simulink model "NodoseNeuron"  (Simulink 7.0)
settings: Solver=ode45  StartTime=0.0  StopTime=1000  MaxStep=20  RelTol=1e-3
InitFcn:
  | T=310.0;       % K
  | R=8.3145;     % J/mole/K or V*C/mol/K
  | F=96485.0;    % C/mole
  | Nai=8.9;         % mM
  | Nao=154;       % mM
  | Ki=145;           % mM
  | Ko=5.4;           % mM
  | Cai=0.0001;    %mM
  | Cao=2.0;         %mM
  | %Cli Clo
  | %Hi Ho
  | %Cli Clo
  | 
  | ENa=R*T/F*log(Nao/Nai)*1000;    % mV
  | EK=R*T/F*log(Ko/Ki)*1000;           % mM
  | ECa=R*T/2/F*log(Cao/Cai)*1000; % mV
  | %EH=R*T/F*log(Ho/Hi)*1000;
  | %ECl=R*T//F*log(Clo/Cli)*1000;
  | 
  | tauCa=4511.0;   % ms
  | nBi=0.004;         % mM (concentration of Ca2+ buffer) * (number of Ca2+ binding sights)
  | Voli=0.0127;      % nl
  | Vols=0.00146;   % nl
  | 
  | ICaP=0.0243;          % nA
  | INaK=0.275;            % nA
  | DNaCa=0.0036;      % 1/mM^4
  | KNaCa=0.000036;  % nA/mM^4
  | KMCaP=0.0005;     % mM
  | KMNa=5.46;           % mM
  | KMK=0.621;            % mM
  | kU=100.0;               % 1/mM/ms
  | kR=0.238;               % 1/ms
undefined symbols (not defined in the file): sigbuilder_block
settings Model: Creator=Vlad  LastModifiedBy=snitsarevv  ExtModeAutoUpdateStatusClock=off  TunableVars=gA,gBCa,gBNa,gCan,gCat,gD,gK,gKCa,gNaf,gNas  TunableVarsStorageClass=Auto,Auto,Auto,Auto,Auto,Auto,Auto,Auto,Auto,Auto  TunableVarsTypeQualifier=,,,,,,,,,  BufferReuse=off
settings SolverCC: ZeroCrossControl=DisableAll
settings DataIOCC: ExternalInput=[t u]  LimitDataPoints=off
settings OptimizationCC: InlineParams=on  OptimizeBlockIOStorage=off  BufferReuse=off  ExpressionFolding=off  LocalBlockOutputs=off
settings DebuggingCC: SaveWithParameterizedLinksMsg=none
settings GRTTargetCC: TargetFcnLib=ansi_tfl_tmw.mat

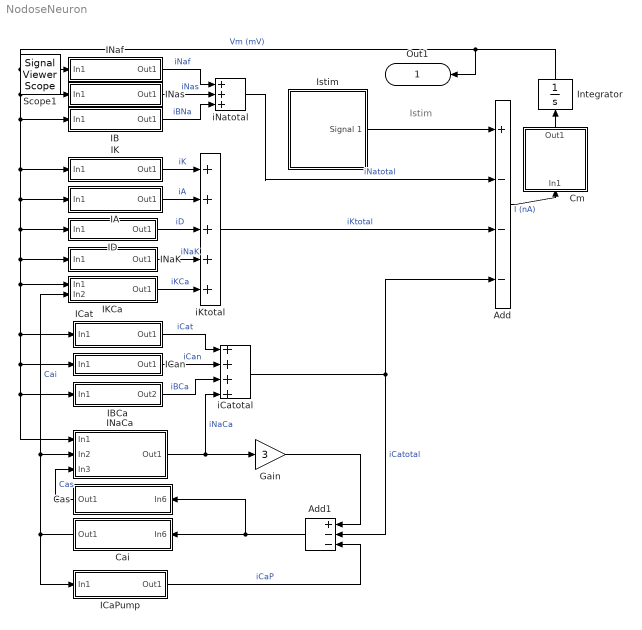
== system NodoseNeuron ==
  note: Istim
  Add : Sum  Inputs=+---  OutDataType=sfix(16)  OutScaling=2^-10
  Add1 : Sum  Orientation=left  Inputs=+--  OutDataType=sfix(16)  OutScaling=2^-10
  Cai : Subsystem  Orientation=left
  Cas : Subsystem  Orientation=left
  Cm : Subsystem  Orientation=up  mask{Cm=32.5}
      mask help: Cm=32.5 pF
  Gain : Gain  Gain=3  ParameterDataType=sfix(16)  ParameterScaling=2^0  OutDataType=sfix(16)  OutScaling=2^0
  IA : Subsystem  mask{gA=0.035}
      mask help: gA=0.035 microS
      mask init:
      | %gA=0.035 in SK model
  IB : Subsystem  mask{gBNa=0.000325}
      mask help: gBNa=0.000325 microS
  IBCa : Subsystem  mask{gBCa=0.000085}
      mask help: gBCa=0.000085 microS
  ICaPump : Subsystem
  ICan : Subsystem  mask{gCan=0.001}
      mask help: gCan=0.001 microS
  ICat : Subsystem  mask{gCat=0.00035}
      mask help: gCat=0.00035 microS
  ID : Subsystem  mask{gD=0.01}
      mask help: gD=0.01 microS
  IK : Subsystem  mask{gK=0.0055}
      mask help: gK=0.0055 microS
  IKCa : Subsystem  mask{gKCa=0.0065}
      mask help: gKCa=0.0065 microS
  INaCa : Subsystem
  INaK : Subsystem
  INaf : Subsystem  mask{gNaf=2.05}
      mask help: gNaf=2.05 microS
  INas : Subsystem  mask{gNas=0.00001}
      mask help: gNas=0.00001 microS
  Integrator : Integrator  Orientation=up  InitialCondition=-56.34  UpperSaturationLimit=100  LowerSaturationLimit=-100
  Istim : Subsystem  Tag=STV Subsys  LoadFcn=sigbuilder_block('load');  StartFcn=sigbuilder_block('start');  StopFcn=sigbuilder_block('stop');  ClipboardFcn=sigbuilder_block('clipboard');  mask(Sigbuilder block){}
      mask help: Sigbuilder GUI
      mask init:
      | if ~strcmp(get_param(bdroot(gcbh),'SimulationStatus'),'stopped') tuvar = sigbuilder_block('maskInit'); end
      settings: CopyFcn=sigbuilder_block('copy');  DeleteFcn=sigbuilder_block('delete');  ModelCloseFcn=sigbuilder_block('modelClose');  PreSaveFcn=sigbuilder_block('preSave');  NameChangeFcn=sigbuilder_block('namechange');  OpenFcn=sigbuilder_block('open',[293.25 508.5 663.75 206.25 ]);  CloseFcn=sigbuilder_block('close');
      mask Display: plot(0,0,100,100,[10,10,40,40,10],[80,20,20,80,80],[40,10],[50,50], [40,27,10],[65,72,56],[40,25,25,10],[28,28,43,43]);
  iCatotal : Sum  Inputs=++++  OutDataType=sfix(16)  OutScaling=2^-10
  iKtotal : Sum  Inputs=+++++  OutDataType=sfix(16)  OutScaling=2^-10
  iNatotal : Sum  Inputs=+++  OutDataType=sfix(16)  OutScaling=2^-10
  Out1 : Outport  Orientation=left  OutDataType=sfix(16)  OutScaling=2^0
  Scope1 : SignalViewerScope  IOType=viewer  LegendLocations="567.3333           436            97      20.33333"  RefreshTime=0.035000
      settings: ShowLegends=on  TimeRange=1000  YMin=-80  YMax=80
  wires:
  Cm/1(Out1) -> Integrator/1
  Add/1 -> Cm/1(In1)  "I (nA)"
  INaf/1(Out1) -> iNatotal/1  "iNaf"
  INas/1(Out1) -> iNatotal/2  "iNas"
  IK/1(Out1) -> iKtotal/1  "iK"
  IA/1(Out1) -> iKtotal/2  "iA"
  ID/1(Out1) -> iKtotal/3  "iD"
  INaK/1(Out1) -> iKtotal/4  "iNaK"
  Cas/1(Out1) -> INaCa/3(In3)  "Cas"
  Cai/1(Out1) -> INaCa/2(In2), IKCa/2(In2), ICaPump/1(In1)  "Cai"
  IKCa/1(Out1) -> iKtotal/5  "iKCa"
  IB/1(Out1) -> iNatotal/3  "iBNa"
  ICat/1(Out1) -> iCatotal/1  "iCat"
  ICan/1(Out1) -> iCatotal/2  "iCan"
  iCatotal/1 -> Add1/2, Add/4  "iCatotal"
  ICaPump/1(Out1) -> Add1/3  "iCaP"
  INaCa/1(Out1) -> iCatotal/4, Gain/1  "iNaCa"
  Add1/1 -> Cas/1(In6), Cai/1(In6)
  Gain/1 -> Add1/1
  iKtotal/1 -> Add/3  "iKtotal"
  iNatotal/1 -> Add/2  "iNatotal"
  Integrator/1 -> Out1/1, INaf/1(In1), INas/1(In1), IB/1(In1), IA/1(In1), ID/1(In1), INaK/1(In1), IBCa/1(In1), INaCa/1(In1), ICan/1(In1), ICat/1(In1), IKCa/1(In1), IK/1(In1)  "Vm (mV)"
  Istim/1(Signal 1) -> Add/1
  IBCa/1(Out2) -> iCatotal/3  "iBCa"

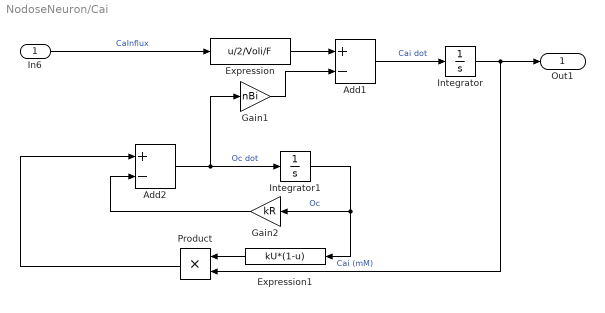
== system NodoseNeuron/Cai ==
  In6 : Inport  OutDataType=sfix(16)  OutScaling=2^0
  Add1 : Sum  Inputs=+-  OutDataType=sfix(16)  OutScaling=2^-10
  Add2 : Sum  Inputs=+-  OutDataType=sfix(16)  OutScaling=2^-10
  Expression : Fcn  Expr=u/2/Voli/F
  Expression1 : Fcn  Orientation=left  Expr=kU*(1-u)
  Gain1 : Gain  Gain=nBi  ParameterDataType=sfix(16)  ParameterScaling=2^0  OutDataType=sfix(16)  OutScaling=2^0
  Gain2 : Gain  Orientation=left  Gain=kR  ParameterDataType=sfix(16)  ParameterScaling=2^0  OutDataType=sfix(16)  OutScaling=2^0
  Integrator : Integrator  InitialCondition=0.00008424  LimitOutput=on  UpperSaturationLimit=0.001  LowerSaturationLimit=0
  Integrator1 : Integrator  InitialCondition=0.03418  LimitOutput=on  UpperSaturationLimit=1  LowerSaturationLimit=0
  Product : Product  Orientation=left  OutDataType=sfix(16)  OutScaling=2^0  RndMeth=Zero
  Out1 : Outport  OutDataType=sfix(16)  OutScaling=2^0
  wires:
  Add1/1 -> Integrator/1  "Cai dot"
  Integrator/1 -> Out1/1, Product/2  "Cai (mM)"
  In6/1 -> Expression/1  "CaInflux"
  Expression/1 -> Add1/1
  Add2/1 -> Integrator1/1, Gain1/1  "Oc dot"
  Gain1/1 -> Add1/2
  Integrator1/1 -> Expression1/1, Gain2/1  "Oc"
  Expression1/1 -> Product/1
  Product/1 -> Add2/1
  Gain2/1 -> Add2/2

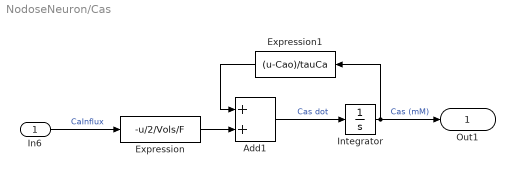
== system NodoseNeuron/Cas ==
  In6 : Inport  OutDataType=sfix(16)  OutScaling=2^0
  Add1 : Sum  OutDataType=sfix(16)  OutScaling=2^-10
  Expression : Fcn  Expr=-u/2/Vols/F
  Expression1 : Fcn  Orientation=left  Expr=(u-Cao)/tauCa
  Integrator : Integrator  InitialCondition=1.7131  LimitOutput=on  UpperSaturationLimit=2  LowerSaturationLimit=0
  Out1 : Outport  OutDataType=sfix(16)  OutScaling=2^0
  wires:
  In6/1 -> Expression/1  "CaInflux"
  Integrator/1 -> Expression1/1, Out1/1  "Cas (mM)"
  Expression1/1 -> Add1/1
  Add1/1 -> Integrator/1  "Cas dot"
  Expression/1 -> Add1/2

== system NodoseNeuron/Cm ==
  In1 : Inport  Orientation=up  OutDataType=sfix(16)  OutScaling=2^0
  Cm : Fcn  Orientation=up  Expr=u/Cm*1000.0
  Out1 : Outport  Orientation=up  OutDataType=sfix(16)  OutScaling=2^0
  wires:
  Cm/1 -> Out1/1  "Vm dot"
  In1/1 -> Cm/1

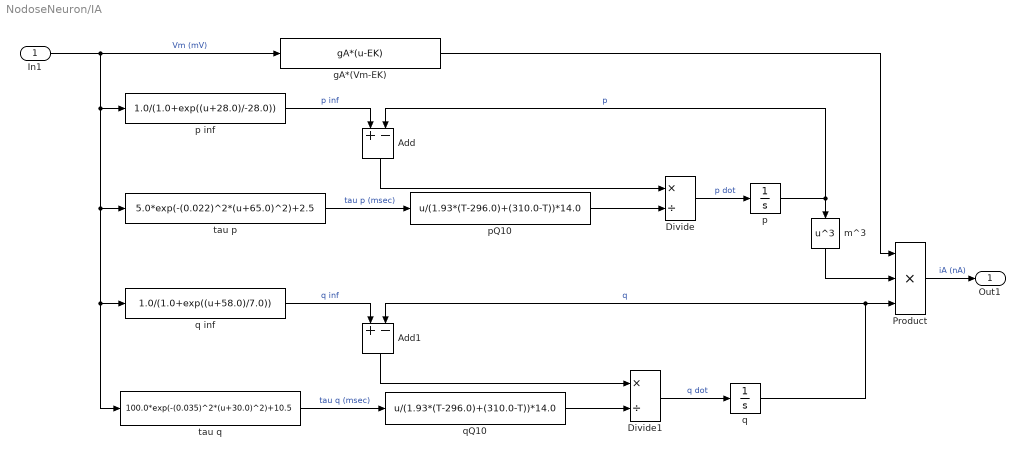
== system NodoseNeuron/IA ==
  In1 : Inport  OutDataType=sfix(16)  OutScaling=2^0
  Add : Sum  Orientation=down  Inputs=+-  OutDataType=sfix(16)  OutScaling=2^-10
  Add1 : Sum  Orientation=down  Inputs=+-  OutDataType=sfix(16)  OutScaling=2^-10
  Divide : Product  Inputs=*/  OutDataType=sfix(16)  OutScaling=2^-10
  Divide1 : Product  Inputs=*/  OutDataType=sfix(16)  OutScaling=2^-10
  Product : Product  Inputs=3  OutDataType=sfix(16)  OutScaling=2^0  RndMeth=Zero
  gA*(Vm-EK) : Fcn  Expr=gA*(u-EK)
  m^3 : Fcn  Orientation=down  Expr=u^3
  p : Integrator  InitialCondition=0.2866  LimitOutput=on  UpperSaturationLimit=1  LowerSaturationLimit=0
  p inf : Fcn  Expr=1.0/(1.0+exp((u+28.0)/-28.0))
  pQ10 : Fcn  Expr=u/(1.93*(T-296.0)+(310.0-T))*14.0
  q : Integrator  InitialCondition=0.3455  LimitOutput=on  UpperSaturationLimit=1  LowerSaturationLimit=0
  q inf : Fcn  Expr=1.0/(1.0+exp((u+58.0)/7.0))
  qQ10 : Fcn  Expr=u/(1.93*(T-296.0)+(310.0-T))*14.0
  tau p : Fcn  Expr=5.0*exp(-(0.022)^2*(u+65.0)^2)+2.5
  tau q : Fcn  Expr=100.0*exp(-(0.035)^2*(u+30.0)^2)+10.5
  Out1 : Outport  OutDataType=sfix(16)  OutScaling=2^0  InitialOutput=0
  wires:
  In1/1 -> q inf/1, tau q/1, tau p/1, p inf/1, gA*(Vm-EK)/1  "Vm (mV)"
  p inf/1 -> Add/1  "p inf"
  p/1 -> m^3/1, Add/2  "p"
  tau p/1 -> pQ10/1  "tau p (msec)"
  Add/1 -> Divide/1
  Divide/1 -> p/1  "p dot"
  q inf/1 -> Add1/1  "q inf"
  Divide1/1 -> q/1  "q dot"
  Add1/1 -> Divide1/1
  tau q/1 -> qQ10/1  "tau q (msec)"
  q/1 -> Add1/2, Product/3  "q"
  Product/1 -> Out1/1  "iA (nA)"
  pQ10/1 -> Divide/2
  qQ10/1 -> Divide1/2
  gA*(Vm-EK)/1 -> Product/1
  m^3/1 -> Product/2

== system NodoseNeuron/IB ==
  In1 : Inport  OutDataType=sfix(16)  OutScaling=2^0
  IBNa : Fcn  Expr=gBNa*(u-ENa)
  Out1 : Outport  OutDataType=sfix(16)  OutScaling=2^0  InitialOutput=0
  wires:
  IBNa/1 -> Out1/1  "iBNa (nA)"
  In1/1 -> IBNa/1  "Vm (mV)"

== system NodoseNeuron/IBCa ==
  In1 : Inport  OutDataType=sfix(16)  OutScaling=2^0
  IBCa : Fcn  Expr=gBCa*(u-ECa)
  Out2 : Outport  OutDataType=sfix(16)  OutScaling=2^0  InitialOutput=0
  wires:
  In1/1 -> IBCa/1  "Vm (mV)"
  IBCa/1 -> Out2/1  "iBCa"

== system NodoseNeuron/ICaPump ==
  In1 : Inport  OutDataType=sfix(16)  OutScaling=2^0
  Bias : Bias  Bias=KMCaP
  Divide : Product  Inputs=**/  OutDataType=sfix(16)  OutScaling=2^-10
  Q10 : Constant  Value=ICaP*(2.3*(T-296.0)+(310.0-T))/14.0  OutDataType=sfix(16)  OutScaling=2^0
  Out1 : Outport  OutDataType=sfix(16)  OutScaling=2^0
  wires:
  Bias/1 -> Divide/3
  Divide/1 -> Out1/1  "iCaP"
  In1/1 -> Bias/1, Divide/2  "Cai"
  Q10/1 -> Divide/1

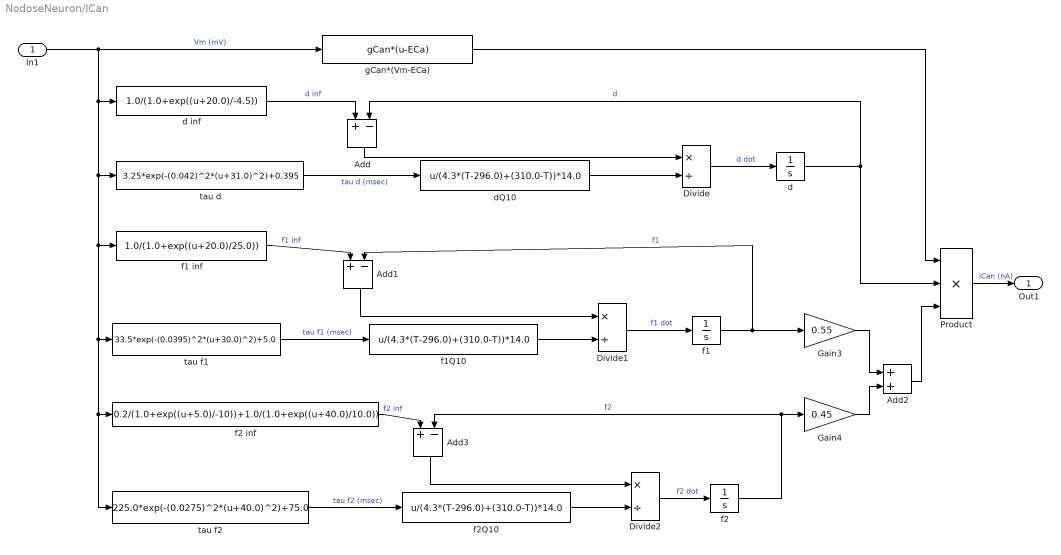
== system NodoseNeuron/ICan ==
  In1 : Inport  OutDataType=sfix(16)  OutScaling=2^0
  Add : Sum  Orientation=down  Inputs=+-  OutDataType=sfix(16)  OutScaling=2^-10
  Add1 : Sum  Orientation=down  Inputs=+-  OutDataType=sfix(16)  OutScaling=2^-10
  Add2 : Sum  OutDataType=sfix(16)  OutScaling=2^-10
  Add3 : Sum  Orientation=down  Inputs=+-  OutDataType=sfix(16)  OutScaling=2^-10
  Divide : Product  Inputs=*/  OutDataType=sfix(16)  OutScaling=2^-10
  Divide1 : Product  Inputs=*/  OutDataType=sfix(16)  OutScaling=2^-10
  Divide2 : Product  Inputs=*/  OutDataType=sfix(16)  OutScaling=2^-10
  Gain3 : Gain  Gain=0.55  ParameterDataType=sfix(16)  ParameterScaling=2^0  OutDataType=sfix(16)  OutScaling=2^0
  Gain4 : Gain  Gain=0.45  ParameterDataType=sfix(16)  ParameterScaling=2^0  OutDataType=sfix(16)  OutScaling=2^0
  Product : Product  Inputs=3  OutDataType=sfix(16)  OutScaling=2^0  RndMeth=Zero
  d : Integrator  InitialCondition=0.0006  LimitOutput=on  UpperSaturationLimit=1  LowerSaturationLimit=0
  d inf : Fcn  Expr=1.0/(1.0+exp((u+20.0)/-4.5))
  dQ10 : Fcn  Expr=u/(4.3*(T-296.0)+(310.0-T))*14.0
  f1 : Integrator  InitialCondition=0.7927  LimitOutput=on  UpperSaturationLimit=1  LowerSaturationLimit=0
  f1 inf : Fcn  Expr=1.0/(1.0+exp((u+20.0)/25.0))
  f1Q10 : Fcn  Expr=u/(4.3*(T-296.0)+(310.0-T))*14.0
  f2 : Integrator  InitialCondition=0.7962  LimitOutput=on  UpperSaturationLimit=1  LowerSaturationLimit=0
  f2 inf : Fcn  Expr=0.2/(1.0+exp((u+5.0)/-10))+1.0/(1.0+exp((u+40.0)/10.0))
  f2Q10 : Fcn  Expr=u/(4.3*(T-296.0)+(310.0-T))*14.0
  gCan*(Vm-ECa) : Fcn  Expr=gCan*(u-ECa)
  tau d : Fcn  Expr=3.25*exp(-(0.042)^2*(u+31.0)^2)+0.395
  tau f1 : Fcn  Expr=33.5*exp(-(0.0395)^2*(u+30.0)^2)+5.0
  tau f2 : Fcn  Expr=225.0*exp(-(0.0275)^2*(u+40.0)^2)+75.0
  Out1 : Outport  OutDataType=sfix(16)  OutScaling=2^0  InitialOutput=0
  wires:
  In1/1 -> tau d/1, f1 inf/1, tau f1/1, f2 inf/1, tau f2/1, d inf/1, gCan*(Vm-ECa)/1  "Vm (mV)"
  d inf/1 -> Add/1  "d inf"
  d/1 -> Add/2, Product/2  "d"
  tau d/1 -> dQ10/1  "tau d (msec)"
  Add/1 -> Divide/1
  Divide/1 -> d/1  "d dot"
  f1 inf/1 -> Add1/1  "f1 inf"
  Divide1/1 -> f1/1  "f1 dot"
  Add1/1 -> Divide1/1
  tau f1/1 -> f1Q10/1  "tau f1 (msec)"
  f1/1 -> Gain3/1, Add1/2  "f1"
  Product/1 -> Out1/1  "iCan (nA)"
  f2 inf/1 -> Add3/1  "f2 inf"
  Divide2/1 -> f2/1  "f2 dot"
  Add3/1 -> Divide2/1
  tau f2/1 -> f2Q10/1  "tau f2 (msec)"
  Gain3/1 -> Add2/1
  Gain4/1 -> Add2/2
  f2/1 -> Gain4/1, Add3/2  "f2"
  dQ10/1 -> Divide/2
  f1Q10/1 -> Divide1/2
  f2Q10/1 -> Divide2/2
  Add2/1 -> Product/3
  gCan*(Vm-ECa)/1 -> Product/1

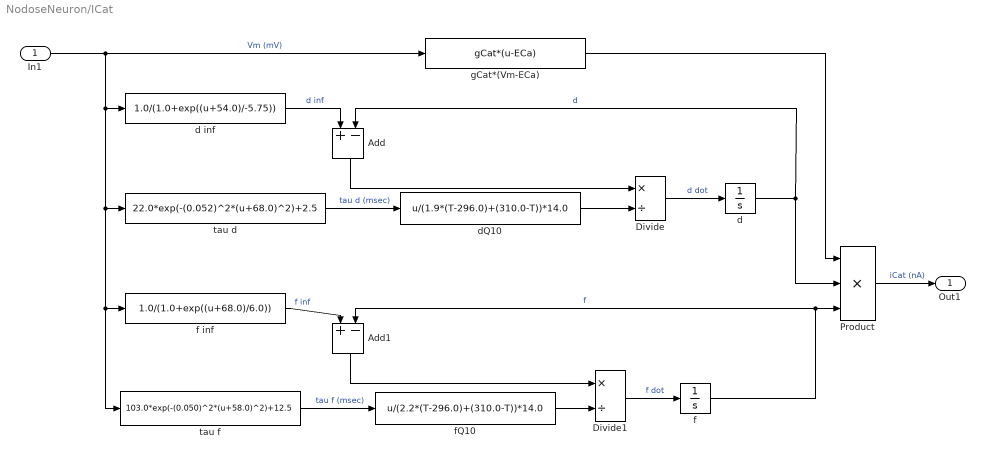
== system NodoseNeuron/ICat ==
  In1 : Inport  OutDataType=sfix(16)  OutScaling=2^0
  Add : Sum  Orientation=down  Inputs=+-  OutDataType=sfix(16)  OutScaling=2^-10
  Add1 : Sum  Orientation=down  Inputs=+-  OutDataType=sfix(16)  OutScaling=2^-10
  Divide : Product  Inputs=*/  OutDataType=sfix(16)  OutScaling=2^-10
  Divide1 : Product  Inputs=*/  OutDataType=sfix(16)  OutScaling=2^-10
  Product : Product  Inputs=3  OutDataType=sfix(16)  OutScaling=2^0  RndMeth=Zero
  d : Integrator  InitialCondition=0.5205  LimitOutput=on  UpperSaturationLimit=1  LowerSaturationLimit=0
  d inf : Fcn  Expr=1.0/(1.0+exp((u+54.0)/-5.75))
  dQ10 : Fcn  Expr=u/(1.9*(T-296.0)+(310.0-T))*14.0
  f : Integrator  InitialCondition=0.0823  LimitOutput=on  UpperSaturationLimit=1  LowerSaturationLimit=0
  f inf : Fcn  Expr=1.0/(1.0+exp((u+68.0)/6.0))
  fQ10 : Fcn  Expr=u/(2.2*(T-296.0)+(310.0-T))*14.0
  gCat*(Vm-ECa) : Fcn  Expr=gCat*(u-ECa)
  tau d : Fcn  Expr=22.0*exp(-(0.052)^2*(u+68.0)^2)+2.5
  tau f : Fcn  Expr=103.0*exp(-(0.050)^2*(u+58.0)^2)+12.5
  Out1 : Outport  OutDataType=sfix(16)  OutScaling=2^0  InitialOutput=0
  wires:
  In1/1 -> f inf/1, tau f/1, tau d/1, d inf/1, gCat*(Vm-ECa)/1  "Vm (mV)"
  d inf/1 -> Add/1  "d inf"
  d/1 -> Add/2, Product/2  "d"
  tau d/1 -> dQ10/1  "tau d (msec)"
  Add/1 -> Divide/1
  Divide/1 -> d/1  "d dot"
  f inf/1 -> Add1/1  "f inf"
  Divide1/1 -> f/1  "f dot"
  Add1/1 -> Divide1/1
  tau f/1 -> fQ10/1  "tau f (msec)"
  f/1 -> Add1/2, Product/3  "f"
  Product/1 -> Out1/1  "iCat (nA)"
  dQ10/1 -> Divide/2
  fQ10/1 -> Divide1/2
  gCat*(Vm-ECa)/1 -> Product/1

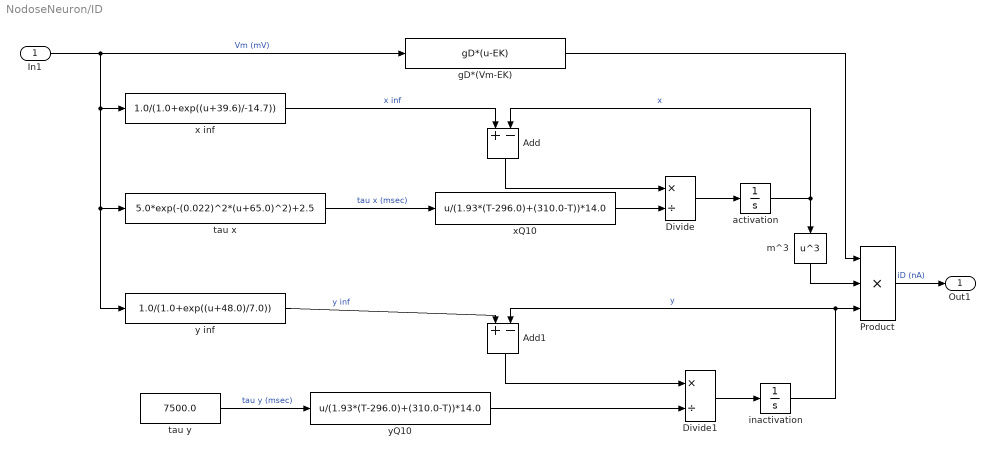
== system NodoseNeuron/ID ==
  In1 : Inport  OutDataType=sfix(16)  OutScaling=2^0
  Add : Sum  Orientation=down  Inputs=+-  OutDataType=sfix(16)  OutScaling=2^-10
  Add1 : Sum  Orientation=down  Inputs=+-  OutDataType=sfix(16)  OutScaling=2^-10
  Divide : Product  Inputs=*/  OutDataType=sfix(16)  OutScaling=2^-10
  Divide1 : Product  Inputs=*/  OutDataType=sfix(16)  OutScaling=2^-10
  Product : Product  Inputs=3  OutDataType=sfix(16)  OutScaling=2^0  RndMeth=Zero
  activation : Integrator  InitialCondition=0.2794  LimitOutput=on  UpperSaturationLimit=1  LowerSaturationLimit=0
  gD*(Vm-EK) : Fcn  Expr=gD*(u-EK)
  inactivation : Integrator  InitialCondition=0.7162  LimitOutput=on  UpperSaturationLimit=1  LowerSaturationLimit=0
  m^3 : Fcn  Orientation=down  Expr=u^3
  tau x : Fcn  Expr=5.0*exp(-(0.022)^2*(u+65.0)^2)+2.5
  tau y : Constant  Value=7500.0  OutDataType=sfix(16)  OutScaling=2^0
  x inf : Fcn  Expr=1.0/(1.0+exp((u+39.6)/-14.7))
  xQ10 : Fcn  Expr=u/(1.93*(T-296.0)+(310.0-T))*14.0
  y inf : Fcn  Expr=1.0/(1.0+exp((u+48.0)/7.0))
  yQ10 : Fcn  Expr=u/(1.93*(T-296.0)+(310.0-T))*14.0
  Out1 : Outport  OutDataType=sfix(16)  OutScaling=2^0
  wires:
  In1/1 -> tau x/1, y inf/1, x inf/1, gD*(Vm-EK)/1  "Vm (mV)"
  x inf/1 -> Add/1  "x inf"
  activation/1 -> m^3/1, Add/2  "x"
  tau x/1 -> xQ10/1  "tau x (msec)"
  Add/1 -> Divide/1
  Divide/1 -> activation/1
  y inf/1 -> Add1/1  "y inf"
  Divide1/1 -> inactivation/1
  Add1/1 -> Divide1/1
  tau y/1 -> yQ10/1  "tau y (msec)"
  inactivation/1 -> Add1/2, Product/3  "y"
  Product/1 -> Out1/1  "iD (nA)"
  xQ10/1 -> Divide/2
  yQ10/1 -> Divide1/2
  m^3/1 -> Product/2
  gD*(Vm-EK)/1 -> Product/1

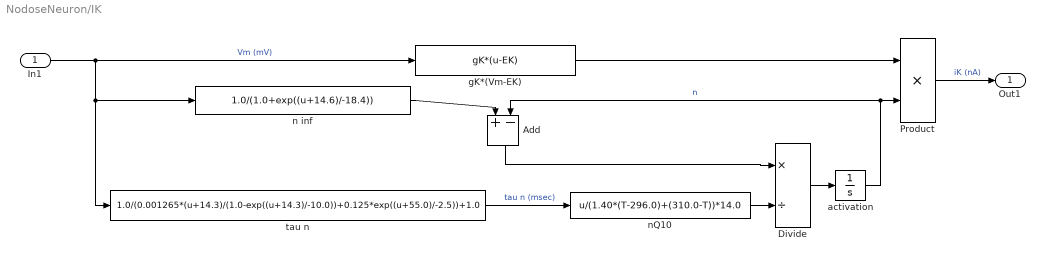
== system NodoseNeuron/IK ==
  In1 : Inport  OutDataType=sfix(16)  OutScaling=2^0
  Add : Sum  Orientation=down  Inputs=+-  OutDataType=sfix(16)  OutScaling=2^-10
  Divide : Product  Inputs=*/  OutDataType=sfix(16)  OutScaling=2^-10
  Product : Product  OutDataType=sfix(16)  OutScaling=2^0  RndMeth=Zero
  activation : Integrator  InitialCondition=0.1076  LimitOutput=on  UpperSaturationLimit=1  LowerSaturationLimit=0
  gK*(Vm-EK) : Fcn  Expr=gK*(u-EK)
  n inf : Fcn  Expr=1.0/(1.0+exp((u+14.6)/-18.4))
  nQ10 : Fcn  Expr=u/(1.40*(T-296.0)+(310.0-T))*14.0
  tau n : Fcn  Expr=1.0/(0.001265*(u+14.3)/(1.0-exp((u+14.3)/-10.0))+0.125*exp((u+55.0)/-2.5))+1.0
  Out1 : Outport  OutDataType=sfix(16)  OutScaling=2^0  InitialOutput=0
  wires:
  n inf/1 -> Add/1
  tau n/1 -> nQ10/1  "tau n (msec)"
  Add/1 -> Divide/1
  Divide/1 -> activation/1
  Product/1 -> Out1/1  "iK (nA)"
  activation/1 -> Add/2, Product/2  "n"
  In1/1 -> n inf/1, tau n/1, gK*(Vm-EK)/1  "Vm (mV)"
  nQ10/1 -> Divide/2
  gK*(Vm-EK)/1 -> Product/1

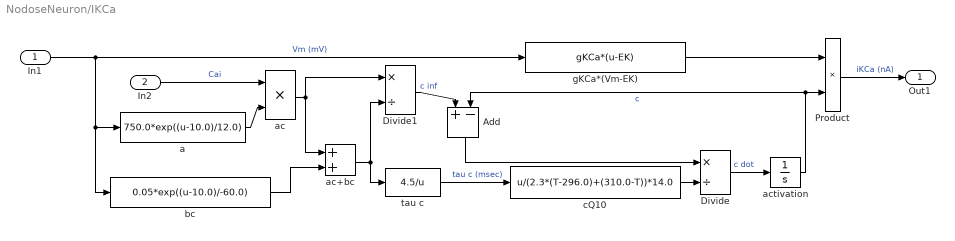
== system NodoseNeuron/IKCa ==
  In1 : Inport  OutDataType=sfix(16)  OutScaling=2^0
  In2 : Inport  Port=2  OutDataType=sfix(16)  OutScaling=2^0
  Add : Sum  Orientation=down  Inputs=+-  OutDataType=sfix(16)  OutScaling=2^-10
  Divide : Product  Inputs=*/  OutDataType=sfix(16)  OutScaling=2^-10
  Divide1 : Product  Inputs=*/  OutDataType=sfix(16)  OutScaling=2^-10
  Product : Product  OutDataType=sfix(16)  OutScaling=2^0  RndMeth=Zero
  a : Fcn  Expr=750.0*exp((u-10.0)/12.0)
  ac : Product  Inputs=**  OutDataType=sfix(16)  OutScaling=2^-10
  ac+bc : Sum  OutDataType=sfix(16)  OutScaling=2^-10
  activation : Integrator  InitialCondition=0.0046  LimitOutput=on  UpperSaturationLimit=1  LowerSaturationLimit=0
  bc : Fcn  Expr=0.05*exp((u-10.0)/-60.0)
  cQ10 : Fcn  Expr=u/(2.3*(T-296.0)+(310.0-T))*14.0
  gKCa*(Vm-EK) : Fcn  Expr=gKCa*(u-EK)
  tau c : Fcn  Expr=4.5/u
  Out1 : Outport  OutDataType=sfix(16)  OutScaling=2^0  InitialOutput=0
  wires:
  In1/1 -> bc/1, a/1, gKCa*(Vm-EK)/1  "Vm (mV)"
  tau c/1 -> cQ10/1  "tau c (msec)"
  Add/1 -> Divide/1
  Divide/1 -> activation/1  "c dot"
  Product/1 -> Out1/1  "iKCa (nA)"
  ac+bc/1 -> Divide1/2, tau c/1
  Divide1/1 -> Add/1  "c inf"
  bc/1 -> ac+bc/2
  a/1 -> ac/2
  ac/1 -> ac+bc/1, Divide1/1
  In2/1 -> ac/1  "Cai"
  cQ10/1 -> Divide/2
  activation/1 -> Add/2, Product/2  "c"
  gKCa*(Vm-EK)/1 -> Product/1

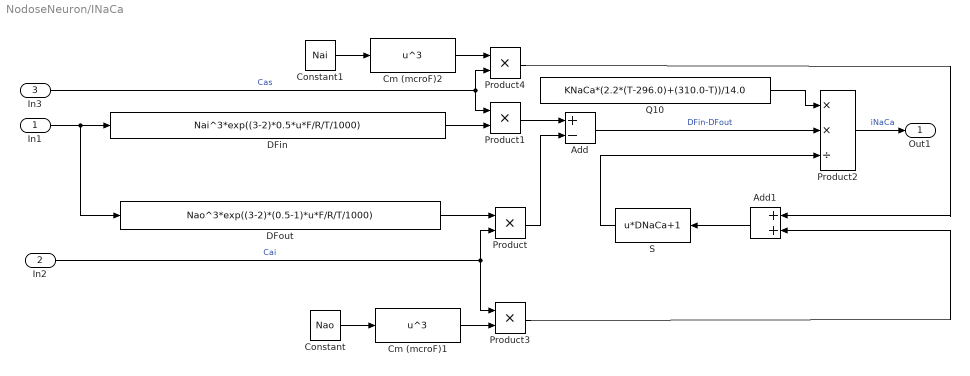
== system NodoseNeuron/INaCa ==
  In1 : Inport  OutDataType=sfix(16)  OutScaling=2^0
  In2 : Inport  Port=2  OutDataType=sfix(16)  OutScaling=2^0
  In3 : Inport  Port=3  OutDataType=sfix(16)  OutScaling=2^0
  Add : Sum  Inputs=+-  OutDataType=sfix(16)  OutScaling=2^-10
  Add1 : Sum  Orientation=left  OutDataType=sfix(16)  OutScaling=2^-10
  Cm (mcroF)1 : Fcn  Expr=u^3
  Cm (mcroF)2 : Fcn  Expr=u^3
  Constant : Constant  Value=Nao  OutDataType=sfix(16)  OutScaling=2^0
  Constant1 : Constant  Value=Nai  VectorParams1D=off  OutDataType=sfix(16)  OutScaling=2^0
  DFin : Fcn  Expr=Nai^3*exp((3-2)*0.5*u*F/R/T/1000)
  DFout : Fcn  Expr=Nao^3*exp((3-2)*(0.5-1)*u*F/R/T/1000)
  Product{,1,3..4} (4 alike) : Product  OutDataType=sfix(16)  OutScaling=2^0  RndMeth=Zero
  Product2 : Product  Inputs=**/  OutDataType=sfix(16)  OutScaling=2^0  RndMeth=Zero
  Q10 : Constant  Value=KNaCa*(2.2*(T-296.0)+(310.0-T))/14.0  OutDataType=sfix(16)  OutScaling=2^0
  S : Fcn  Orientation=left  Expr=u*DNaCa+1
  Out1 : Outport  OutDataType=sfix(16)  OutScaling=2^0
  wires:
  Add/1 -> Product2/2  "DFin-DFout"
  In1/1 -> DFin/1, DFout/1
  Product/1 -> Add/2
  In2/1 -> Product/2, Product3/1  "Cai"
  DFin/1 -> Product1/2
  Product1/1 -> Add/1
  In3/1 -> Product1/1, Product4/2  "Cas"
  DFout/1 -> Product/1
  Constant/1 -> Cm (mcroF)1/1
  Cm (mcroF)1/1 -> Product3/2
  Constant1/1 -> Cm (mcroF)2/1
  Cm (mcroF)2/1 -> Product4/1
  Product4/1 -> Add1/1
  Product3/1 -> Add1/2
  Add1/1 -> S/1
  Product2/1 -> Out1/1  "iNaCa"
  S/1 -> Product2/3
  Q10/1 -> Product2/1

== system NodoseNeuron/INaK ==
  In1 : Inport  OutDataType=sfix(16)  OutScaling=2^0
  INaK : Fcn  Expr=INaK*(Nai/(Nai+KMNa))^3*(Ko/(Ko+KMK))^2*(u+150)/(u+200)
  Product : Product  OutDataType=sfix(16)  OutScaling=2^0  RndMeth=Zero
  Q10 : Constant  Value=(1.16*(T-296.0)+(310.0-T))/14.0  OutDataType=sfix(16)  OutScaling=2^0
  Out1 : Outport  OutDataType=sfix(16)  OutScaling=2^0
  wires:
  In1/1 -> INaK/1  "Vm (mV)"
  INaK/1 -> Product/1
  Q10/1 -> Product/2
  Product/1 -> Out1/1  "iNaK"

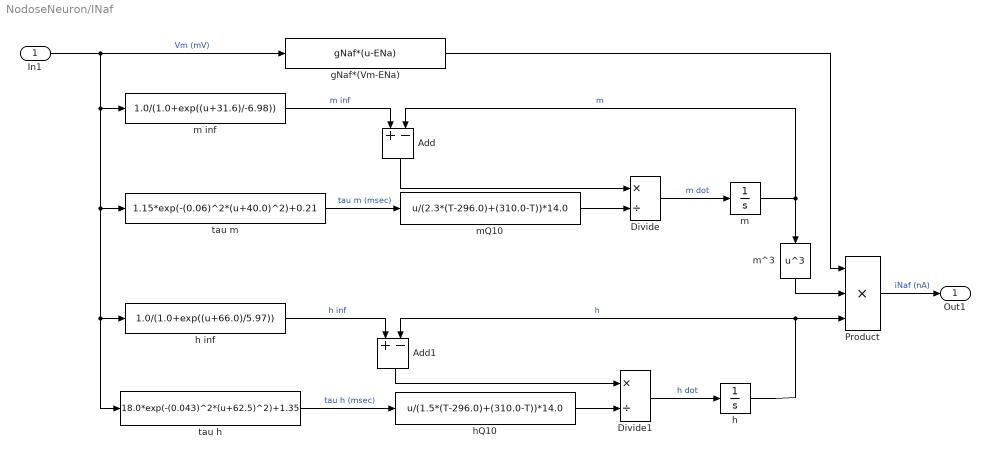
== system NodoseNeuron/INaf ==
  In1 : Inport  OutDataType=sfix(16)  OutScaling=2^0
  Add : Sum  Orientation=down  Inputs=+-  OutDataType=sfix(16)  OutScaling=2^-10
  Add1 : Sum  Orientation=down  Inputs=+-  OutDataType=sfix(16)  OutScaling=2^-10
  Divide : Product  Inputs=*/  OutDataType=sfix(16)  OutScaling=2^-10
  Divide1 : Product  Inputs=*/  OutDataType=sfix(16)  OutScaling=2^-10
  Product : Product  Inputs=3  OutDataType=sfix(16)  OutScaling=2^0  RndMeth=Zero
  gNaf*(Vm-ENa) : Fcn  Expr=gNaf*(u-ENa)
  h : Integrator  InitialCondition=0.1102  LimitOutput=on  UpperSaturationLimit=1  LowerSaturationLimit=0
  h inf : Fcn  Expr=1.0/(1.0+exp((u+66.0)/5.97))
  hQ10 : Fcn  Expr=u/(1.5*(T-296.0)+(310.0-T))*14.0
  m : Integrator  InitialCondition=0.0414  LimitOutput=on  UpperSaturationLimit=1  LowerSaturationLimit=0
  m inf : Fcn  Expr=1.0/(1.0+exp((u+31.6)/-6.98))
  mQ10 : Fcn  Expr=u/(2.3*(T-296.0)+(310.0-T))*14.0
  m^3 : Fcn  Orientation=down  Expr=u^3
  tau h : Fcn  Expr=18.0*exp(-(0.043)^2*(u+62.5)^2)+1.35
  tau m : Fcn  Expr=1.15*exp(-(0.06)^2*(u+40.0)^2)+0.21
  Out1 : Outport  OutDataType=sfix(16)  OutScaling=2^0  InitialOutput=0
  wires:
  In1/1 -> h inf/1, tau h/1, tau m/1, m inf/1, gNaf*(Vm-ENa)/1  "Vm (mV)"
  m inf/1 -> Add/1  "m inf"
  m/1 -> m^3/1, Add/2  "m"
  tau m/1 -> mQ10/1  "tau m (msec)"
  Add/1 -> Divide/1
  Divide/1 -> m/1  "m dot"
  h inf/1 -> Add1/1  "h inf"
  Divide1/1 -> h/1  "h dot"
  Add1/1 -> Divide1/1
  tau h/1 -> hQ10/1  "tau h (msec)"
  h/1 -> Add1/2, Product/3  "h"
  Product/1 -> Out1/1  "iNaf (nA)"
  mQ10/1 -> Divide/2
  hQ10/1 -> Divide1/2
  gNaf*(Vm-ENa)/1 -> Product/1
  m^3/1 -> Product/2

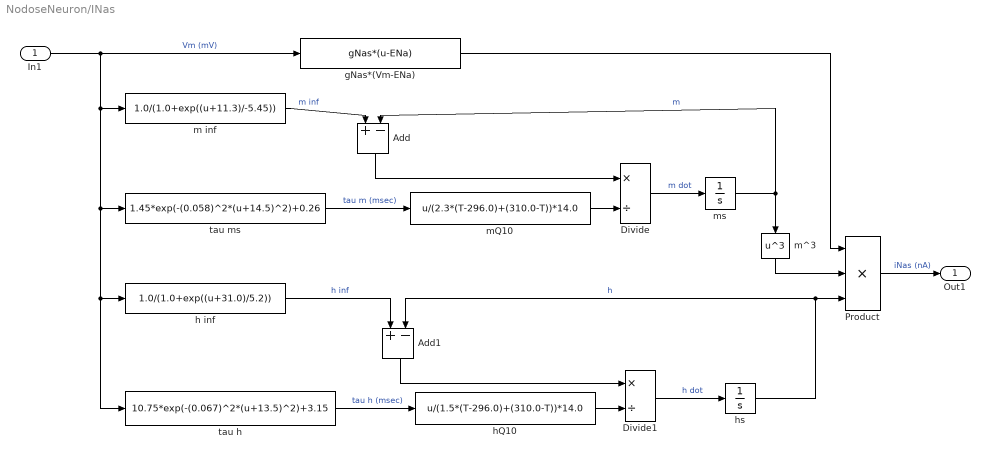
== system NodoseNeuron/INas ==
  In1 : Inport  OutDataType=sfix(16)  OutScaling=2^0
  Add : Sum  Orientation=down  Inputs=+-  OutDataType=sfix(16)  OutScaling=2^-10
  Add1 : Sum  Orientation=down  Inputs=+-  OutDataType=sfix(16)  OutScaling=2^-10
  Divide : Product  Inputs=*/  OutDataType=sfix(16)  OutScaling=2^-10
  Divide1 : Product  Inputs=*/  OutDataType=sfix(16)  OutScaling=2^-10
  Product : Product  Inputs=3  OutDataType=sfix(16)  OutScaling=2^0  RndMeth=Zero
  gNas*(Vm-ENa) : Fcn  Expr=gNas*(u-ENa)
  h inf : Fcn  Expr=1.0/(1.0+exp((u+31.0)/5.2))
  hQ10 : Fcn  Expr=u/(1.5*(T-296.0)+(310.0-T))*14.0
  hs : Integrator  InitialCondition=0.9870  LimitOutput=on  UpperSaturationLimit=1.0  LowerSaturationLimit=0.0
  m inf : Fcn  Expr=1.0/(1.0+exp((u+11.3)/-5.45))
  mQ10 : Fcn  Expr=u/(2.3*(T-296.0)+(310.0-T))*14.0
  m^3 : Fcn  Orientation=down  Expr=u^3
  ms : Integrator  InitialCondition=0.0004  LimitOutput=on  UpperSaturationLimit=1.0  LowerSaturationLimit=0.0
  tau h : Fcn  Expr=10.75*exp(-(0.067)^2*(u+13.5)^2)+3.15
  tau ms : Fcn  Expr=1.45*exp(-(0.058)^2*(u+14.5)^2)+0.26
  Out1 : Outport  OutDataType=sfix(16)  OutScaling=2^0  InitialOutput=0
  wires:
  In1/1 -> h inf/1, tau h/1, tau ms/1, m inf/1, gNas*(Vm-ENa)/1  "Vm (mV)"
  m inf/1 -> Add/1  "m inf"
  ms/1 -> m^3/1, Add/2  "m"
  tau ms/1 -> mQ10/1  "tau m (msec)"
  Add/1 -> Divide/1
  Divide/1 -> ms/1  "m dot"
  h inf/1 -> Add1/1  "h inf"
  Divide1/1 -> hs/1  "h dot"
  Add1/1 -> Divide1/1
  tau h/1 -> hQ10/1  "tau h (msec)"
  hs/1 -> Add1/2, Product/3  "h"
  Product/1 -> Out1/1  "iNas (nA)"
  mQ10/1 -> Divide/2
  hQ10/1 -> Divide1/2
  gNas*(Vm-ENa)/1 -> Product/1
  m^3/1 -> Product/2

== system NodoseNeuron/Istim ==
  Demux : Demux  Tag=STV Demux  Outputs=1
  FromWs : FromWorkspace  Tag=STV FromWs  VariableName=tuvar  SampleTime=0  SigBuilderData=DataTag0  VnvData=DataTag1
      SigBuilderData=|
      | channels.label = 'Signal 1'
      | channels.allXData = {[0 500 500 1000]}
      | channels.allYData = {[0 0 0.04 0.04]}
      | common.afterFinalStr = 'Extrapolate'
      | common.sampleTime = 0
      | dataSet.timeRange = [0 1000]
      | dataSet.name = 'Group 1'
  Signal 1 : Outport  Tag=STV Outport  OutDataType=sfix(16)  OutScaling=2^0
  wires:
  FromWs/1 -> Demux/1
  Demux/1 -> Signal 1/1
